simulink model "observerFeedBack"  (R2019b)
settings: Solver=VariableStepAuto  StartTime=0.0  StopTime=2  RelTol=1e-3
values from neighbouring files (symbols this model uses):
  A_ob = A    [DC_Motor_Analysis.m]
  B_ob = B    [DC_Motor_Analysis.m]
  C_ob = C    [DC_Motor_Analysis.m]
  encGain = (2*pi)/4096    (= 0.00153398078789)    [DC_Motor_Analysis.m]    (also in Part2.m; Part3.m; lqrPoles.mat; robust.mat)
  feedForwardGain = 1/dcGain    [DC_Motor_Analysis.m]
  K = [K1 K2]    [DC_Motor_Analysis.m]    (also in Part3.m = double(linsolve(meatMat, potatoesMat)))
  L = double(linsolve(meatMat, potatoesMat))    [DC_Motor_Analysis.m]
settings Model: Creator=justinf  LastModifiedBy=justinf

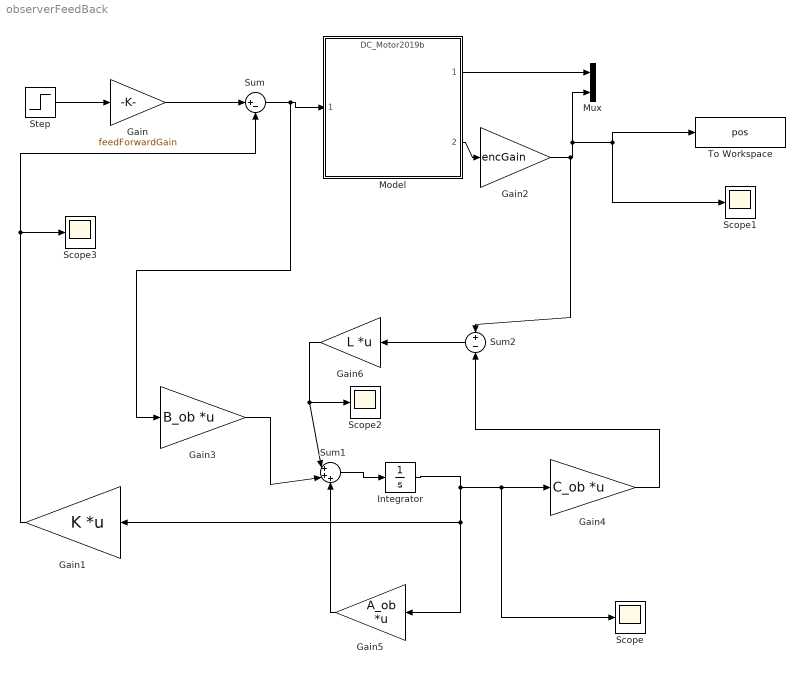
== system observerFeedBack ==
  Gain : Gain  Gain=feedForwardGain
  Gain1 : Gain  Gain=K  Multiplication=Matrix(K*u) (u vector)
  Gain2 : Gain  Gain=encGain
  Gain3 : Gain  Gain=B_ob  Multiplication=Matrix(K*u) (u vector)
  Gain4 : Gain  Gain=C_ob  Multiplication=Matrix(K*u) (u vector)
  Gain5 : Gain  Gain=A_ob  Multiplication=Matrix(K*u) (u vector)
  Gain6 : Gain  Gain=L  Multiplication=Matrix(K*u) (u vector)
  Integrator : Integrator
  Model : ModelReference  ModelNameDialog=DC_Motor2019b.slxp  ModelReferenceVersion=1.20  CopyOfModelProtected=on
  Mux : Mux  Inputs=2
  Scope{,1..3} (4 alike) : Scope
  Step : Step  Time=0  SampleTime=0
  Sum : Sum  Inputs=|+-
  Sum1 : Sum  Inputs=|+++
  Sum2 : Sum  Inputs=+-
  To Workspace : ToWorkspace  VariableName=pos  SampleTime=-1
  wires:
  Model/2 -> Gain2/1
  Gain/1 -> Sum/1
  Gain1/1 -> Scope3/1, Sum/2
  Model/1 -> Mux/1
  Step/1 -> Gain/1
  Gain2/1 -> Sum2/1, Mux/2, Scope1/1, To Workspace/1
  Sum2/1 -> Gain6/1
  Sum1/1 -> Integrator/1
  Integrator/1 -> Gain1/1, Gain5/1, Scope/1, Gain4/1
  Gain4/1 -> Sum2/2
  Sum/1 -> Gain3/1, Model/1
  Gain5/1 -> Sum1/3
  Gain3/1 -> Sum1/2
  Gain6/1 -> Scope2/1, Sum1/1
